simulink model "THERM_FMU"  (R2025b)
settings: Solver=FixedStepAuto  StartTime=0.0  StopTime=20  FixedStep=TsELEC  RelTol=1e-3  AbsTol=1e-6
values from neighbouring files (symbols this model uses):
  TsELEC = 5e-05    [initParams.mat]
  TsTHERMAL = 0.001    [initParams.mat]
undefined symbols (not defined in the file or in its folder): DiscIntNeverNeededParam
libraries: fl_lib x86, nesl_utility x29, SimscapeFluids_lib x4
(part 1 of 2)
Description:
  | Left Actuation System
settings Model: ExtModeAutoUpdateStatusClock=off  Creator=The MathWorks, Inc.  LastModifiedBy=gdudgeon
settings SolverCC: AutoScaleAbsTol=off  AlgebraicLoopSolver=TrustRegion
settings DataIOCC: ExternalInput=[]  InitialState=[]  SaveFormat=Array  SaveOutput=off  SaveTime=off
settings OptimizationCC: BlockReduction=off  BooleanDataType=off  InitFltsAndDblsToZero=on  BufferReusableBoundary=off
settings DebuggingCC: SaveWithParameterizedLinksMsg=none  SignalResolutionControl=TryResolveAllWithWarning  MultiTaskDSMMsg=warning  MultiTaskCondExecSysMsg=none  FcnCallInpInsideContextMsg=warning  UnconnectedInputMsg=warning  UnconnectedOutputMsg=warning  UnconnectedLineMsg=warning  BusObjectLabelMismatch=none  PregeneratedLibrarySubsystemCodeDiagnostic=none  SFUnexpectedBacktrackingDiag=warning  SFNoUnconditionalDefaultTransitionDiag=warning  SFExecutionAtInitializationDiag=none  ArithmeticOperatorsInVariantConditions=warning
settings HardwareCC: ProdBitPerPointer=32.0  ProdBitPerSizeT=32.0  ProdBitPerPtrDiffT=32.0  ProdLargestAtomicFloat=None  ProdIntDivRoundTo=Undefined  ProdEndianess=Unspecified  ProdWordSize=32.0  ProdHWDeviceType=32-bit Generic  TargetUnknown=on
settings ModelReferenceCC: EnableRefExpFcnMdlSchedulingChecks=on  PropagateSignalLabelsOutOfModel=off
settings SFSimCC: SimUseLocalCustomCode=off  CustomCodeUndefinedFunction=UseInterfaceOnly
settings RTWCC: RTWUseLocalCustomCode=off  GPUComputeCapability=3.5
settings CodeAppCC: StateflowObjectComments=on
settings GRTTargetCC: TargetLangStandard=C89/C90 (ANSI)
settings ConfigComp: CovMetricSettings=dw  CovSaveCumulativeToWorkspaceVar=on  CovSaveSingleToWorkspaceVar=on  CovExternalEMLEnable=off

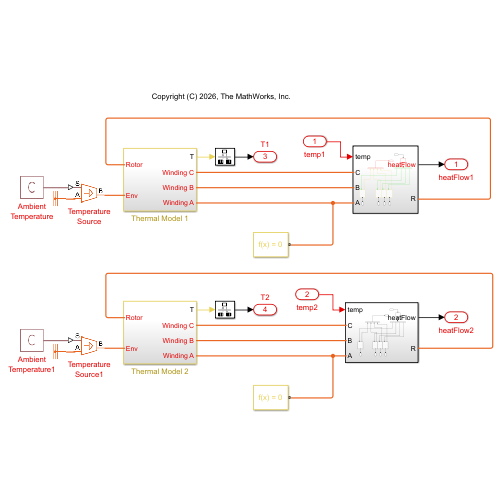
[thumbnail: Simulink's stored preview of the top-level diagram]
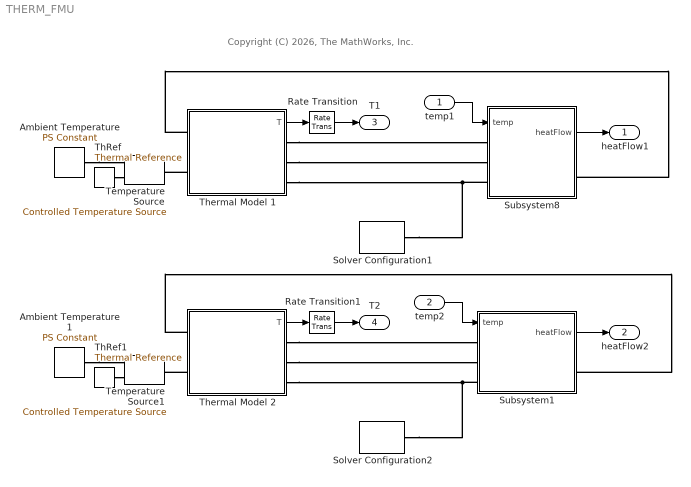
== system THERM_FMU ==
  note: Copyright (C) 2026, The MathWorks, Inc.
  temp1 : Inport  SampleTime=TsELEC
  temp2 : Inport  Port=2  SampleTime=TsELEC
  Ambient Temperature : fl_lib/Physical Signals/Sources/PS Constant  constant=300
  Ambient Temperature1 : fl_lib/Physical Signals/Sources/PS Constant  constant=300
  Rate Transition : RateTransition  OutPortSampleTime=TsELEC
  Rate Transition1 : RateTransition  OutPortSampleTime=TsELEC
  Solver Configuration1 : nesl_utility/Solver Configuration  PhysicalDomain=network_engine_domain  SubClassName=solver  LeftPortType=input  RightPortType=generic  Tones=[]  Harmonics=[]  SimulateNoise=off  Profile=off  UseLocalSampling=off  EnableSwitchedLinearOptims=on  FrequencyDomain=off  UseCCode=off  RelTol=0.001  AbsTol=1e-06  MinStep=1e-09  ToWorkspace=off  RevertToSquareIcSolve=off  NumHomotopyIterations=100  PhasorMode=off  PhasorModeNumHarmonics=1  ConsistencySolver=NEWTON_FTOL  IndexReductionMethod=DerivativeReplacement  DoDC=off  ResidualTolerance=1e-9  ConsistencyTolSource=GLOBAL  ConsistencyAbsTol=0.001  ConsistencyRelTol=0.001  ConsistencyTolFactor=0.001  UseLocalSolver=on  LocalSolverChoice=NE_BACKWARD_EULER_ADVANCER  ResolveIndetEquations=on  FunctionEvalNumThread=1  LocalSolverSampleTime=TsTHERMAL  DoFixedCost=on  MaxNonlinIter=1  MaxModeIter=2  ComputeImpulses=off  ImpulseIterations=2  LinearAlgebra=Full  LinearAlgebraNumThread=0  EquationFormulation=NE_TIME_EF  DelaysMemoryBudget=1024  AutomaticFiltering=on  FilteringTimeConstant=0.001  PartitionStorageMethod=AS_NEEDED  PartitionMemoryBudget=1024  PartitionMethod=FAST  MultibodyUseLocalSolver=off  MultibodyLocalSolverChoice=ODE1  MultibodyLocalSolverSampleTime=0.001
  Solver Configuration2 : nesl_utility/Solver Configuration  PhysicalDomain=network_engine_domain  SubClassName=solver  LeftPortType=input  RightPortType=generic  Tones=[]  Harmonics=[]  SimulateNoise=off  Profile=off  UseLocalSampling=off  EnableSwitchedLinearOptims=on  FrequencyDomain=off  UseCCode=off  RelTol=0.001  AbsTol=1e-06  MinStep=1e-09  ToWorkspace=off  RevertToSquareIcSolve=off  NumHomotopyIterations=100  PhasorMode=off  PhasorModeNumHarmonics=1  ConsistencySolver=NEWTON_FTOL  IndexReductionMethod=DerivativeReplacement  DoDC=off  ResidualTolerance=1e-9  ConsistencyTolSource=GLOBAL  ConsistencyAbsTol=0.001  ConsistencyRelTol=0.001  ConsistencyTolFactor=0.001  UseLocalSolver=on  LocalSolverChoice=NE_BACKWARD_EULER_ADVANCER  ResolveIndetEquations=on  FunctionEvalNumThread=1  LocalSolverSampleTime=TsTHERMAL  DoFixedCost=on  MaxNonlinIter=1  MaxModeIter=2  ComputeImpulses=off  ImpulseIterations=2  LinearAlgebra=Full  LinearAlgebraNumThread=0  EquationFormulation=NE_TIME_EF  DelaysMemoryBudget=1024  AutomaticFiltering=on  FilteringTimeConstant=0.001  PartitionStorageMethod=AS_NEEDED  PartitionMemoryBudget=1024  PartitionMethod=FAST  MultibodyUseLocalSolver=off  MultibodyLocalSolverChoice=ODE1  MultibodyLocalSolverSampleTime=0.001
  Subsystem1 : Subsystem
  Subsystem8 : Subsystem
  Temperature Source : fl_lib/Thermal/Thermal Sources/Controlled Temperature Source
  Temperature Source1 : fl_lib/Thermal/Thermal Sources/Controlled Temperature Source
  ThRef : fl_lib/Thermal/Thermal Elements/Thermal Reference
  ThRef1 : fl_lib/Thermal/Thermal Elements/Thermal Reference
  Thermal Model 1 : Subsystem  Tag=PublishSubsystem
  Thermal Model 2 : Subsystem  Tag=PublishSubsystem
  heatFlow1 : Outport  SampleTime=TsELEC
  heatFlow2 : Outport  Port=2  SampleTime=TsELEC
  T1 : Outport  Port=3  SampleTime=TsELEC
  T2 : Outport  Port=4  SampleTime=TsELEC
  wires:
  Subsystem8/1(heatFlow) -> heatFlow1/1
  temp2/1 -> Subsystem1/1(temp)
  Subsystem1/1(heatFlow) -> heatFlow2/1
  temp1/1 -> Subsystem8/1(temp)
  Thermal Model 1/1(T) -> Rate Transition/1
  Thermal Model 2/1(T) -> Rate Transition1/1
  Rate Transition/1 -> T1/1
  Rate Transition1/1 -> T2/1
  connections:
  Solver Configuration1/RConn1 -- Thermal Model 1/RConn3 -- Subsystem8/LConn3
  Subsystem1/LConn3 -- Thermal Model 2/RConn3 -- Solver Configuration2/RConn1
  ThRef1/LConn1 -- Temperature Source1/RConn2
  Thermal Model 2/RConn1 -- Subsystem1/LConn1
  ThRef/LConn1 -- Temperature Source/RConn2
  Thermal Model 2/LConn1 -- Subsystem1/RConn1
  Thermal Model 1/RConn2 -- Subsystem8/LConn2
  Ambient Temperature1/RConn1 -- Temperature Source1/RConn1
  Ambient Temperature/RConn1 -- Temperature Source/RConn1
  Thermal Model 1/RConn1 -- Subsystem8/LConn1
  Thermal Model 1/LConn1 -- Subsystem8/RConn1
  Thermal Model 2/RConn2 -- Subsystem1/LConn2
  Thermal Model 1/LConn2 -- Temperature Source/LConn1
  Thermal Model 2/LConn2 -- Temperature Source1/LConn1

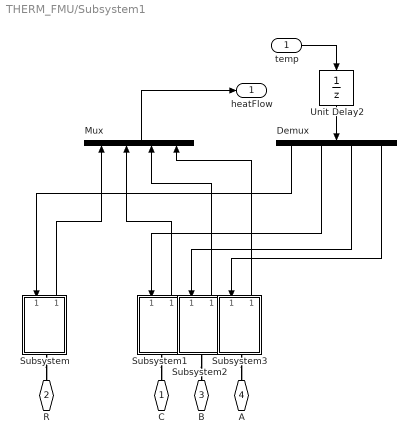
== system THERM_FMU/Subsystem1 ==
  temp : Inport
  Demux : Demux
  Mux : Mux
  Subsystem : Subsystem
      settings: PortSchema="{\"entries\":[{\"content\":{\"sides\":[{\"content\":{\"connectorIds\":[\"LConn1\"]},\"type\":\"ConnectorPlacement.EquallySpacedRectSide\",\"uuid\":\"9a881199-939f-4eef-aa67-0d9d87670dec\"},{\"content\":{\"connectorIds\":[\"In1\",\"Out1\"],\"side\":\"RIGHT\"},\"type\":\"ConnectorPlacement.EquallySpacedRectSide\",\"uuid\":\"59cd7e77-5157-4e0f-8bd7-0ab336b18f97\"},{\"content\":{\"connectorIds\":[],\"side\":\"TOP\"},\"type\":\"ConnectorPlacement.EquallySpacedRectSide\",\"uuid\":\"fe3b6155-18fe-4d88-946d-a6d9bcf9dc7a\"}]},\"type\":\"ConnectorPlacement.EquallySpacedConnector\",\"uuid\":\"f51b1317-3ac5-4211-9ee8-a1dae1b8baeb\"}],\"packageUris\":[\"http://schema.mathworks.com/mf0/Connector/19700101\"],\"version\":\"1.0\"}"
  Subsystem1 : Subsystem
      settings: PortSchema="{\"entries\":[{\"content\":{\"sides\":[{\"content\":{\"connectorIds\":[\"LConn1\"]},\"type\":\"ConnectorPlacement.EquallySpacedRectSide\",\"uuid\":\"9a881199-939f-4eef-aa67-0d9d87670dec\"},{\"content\":{\"connectorIds\":[\"In1\",\"Out1\"],\"side\":\"RIGHT\"},\"type\":\"ConnectorPlacement.EquallySpacedRectSide\",\"uuid\":\"59cd7e77-5157-4e0f-8bd7-0ab336b18f97\"},{\"content\":{\"connectorIds\":[],\"side\":\"TOP\"},\"type\":\"ConnectorPlacement.EquallySpacedRectSide\",\"uuid\":\"fe3b6155-18fe-4d88-946d-a6d9bcf9dc7a\"}]},\"type\":\"ConnectorPlacement.EquallySpacedConnector\",\"uuid\":\"f51b1317-3ac5-4211-9ee8-a1dae1b8baeb\"}],\"packageUris\":[\"http://schema.mathworks.com/mf0/Connector/19700101\"],\"version\":\"1.0\"}"
  Subsystem2 : Subsystem
      settings: PortSchema="{\"entries\":[{\"content\":{\"sides\":[{\"content\":{\"connectorIds\":[\"LConn1\"]},\"type\":\"ConnectorPlacement.EquallySpacedRectSide\",\"uuid\":\"9a881199-939f-4eef-aa67-0d9d87670dec\"},{\"content\":{\"connectorIds\":[\"In1\",\"Out1\"],\"side\":\"RIGHT\"},\"type\":\"ConnectorPlacement.EquallySpacedRectSide\",\"uuid\":\"59cd7e77-5157-4e0f-8bd7-0ab336b18f97\"},{\"content\":{\"connectorIds\":[],\"side\":\"TOP\"},\"type\":\"ConnectorPlacement.EquallySpacedRectSide\",\"uuid\":\"fe3b6155-18fe-4d88-946d-a6d9bcf9dc7a\"}]},\"type\":\"ConnectorPlacement.EquallySpacedConnector\",\"uuid\":\"f51b1317-3ac5-4211-9ee8-a1dae1b8baeb\"}],\"packageUris\":[\"http://schema.mathworks.com/mf0/Connector/19700101\"],\"version\":\"1.0\"}"
  Subsystem3 : Subsystem
      settings: PortSchema="{\"entries\":[{\"content\":{\"sides\":[{\"content\":{\"connectorIds\":[\"LConn1\"]},\"type\":\"ConnectorPlacement.EquallySpacedRectSide\",\"uuid\":\"9a881199-939f-4eef-aa67-0d9d87670dec\"},{\"content\":{\"connectorIds\":[\"In1\",\"Out1\"],\"side\":\"RIGHT\"},\"type\":\"ConnectorPlacement.EquallySpacedRectSide\",\"uuid\":\"59cd7e77-5157-4e0f-8bd7-0ab336b18f97\"},{\"content\":{\"connectorIds\":[],\"side\":\"TOP\"},\"type\":\"ConnectorPlacement.EquallySpacedRectSide\",\"uuid\":\"fe3b6155-18fe-4d88-946d-a6d9bcf9dc7a\"}]},\"type\":\"ConnectorPlacement.EquallySpacedConnector\",\"uuid\":\"f51b1317-3ac5-4211-9ee8-a1dae1b8baeb\"}],\"packageUris\":[\"http://schema.mathworks.com/mf0/Connector/19700101\"],\"version\":\"1.0\"}"
  Unit Delay2 : UnitDelay  InitialCondition=323.15  SampleTime=TsELEC  HasFrameUpgradeWarning=on
  C : PMIOPort  Side=Left
  R : PMIOPort  Port=2  Side=Right
  B : PMIOPort  Port=3  Side=Left
  A : PMIOPort  Port=4  Side=Left
  heatFlow : Outport  SampleTime=TsELEC
  wires:
  temp/1 -> Unit Delay2/1
  Mux/1 -> heatFlow/1
  Subsystem3/1(heatFlow) -> Mux/4
  Demux/4 -> Subsystem3/1(temp)
  Subsystem/1(heatFlow) -> Mux/1
  Demux/1 -> Subsystem/1(temp)
  Unit Delay2/1 -> Demux/1
  Subsystem2/1(heatFlow) -> Mux/3
  Subsystem1/1(heatFlow) -> Mux/2
  Demux/3 -> Subsystem2/1(temp)
  Demux/2 -> Subsystem1/1(temp)
  connections:
  Subsystem1/LConn1 -- C/RConn1
  Subsystem/LConn1 -- R/RConn1
  Subsystem3/LConn1 -- A/RConn1
  Subsystem2/LConn1 -- B/RConn1

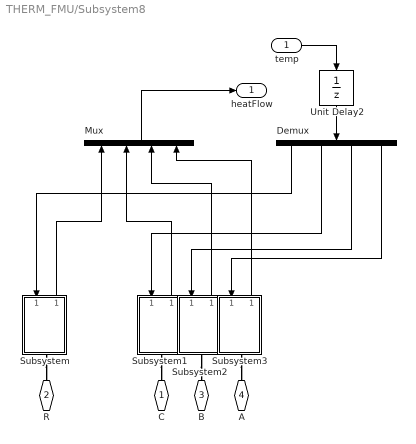
== system THERM_FMU/Subsystem8 ==
  temp : Inport
  Demux : Demux
  Mux : Mux
  Subsystem : Subsystem
      settings: PortSchema="{\"entries\":[{\"content\":{\"sides\":[{\"content\":{\"connectorIds\":[\"LConn1\"]},\"type\":\"ConnectorPlacement.EquallySpacedRectSide\",\"uuid\":\"9a881199-939f-4eef-aa67-0d9d87670dec\"},{\"content\":{\"connectorIds\":[\"In1\",\"Out1\"],\"side\":\"RIGHT\"},\"type\":\"ConnectorPlacement.EquallySpacedRectSide\",\"uuid\":\"59cd7e77-5157-4e0f-8bd7-0ab336b18f97\"},{\"content\":{\"connectorIds\":[],\"side\":\"TOP\"},\"type\":\"ConnectorPlacement.EquallySpacedRectSide\",\"uuid\":\"fe3b6155-18fe-4d88-946d-a6d9bcf9dc7a\"}]},\"type\":\"ConnectorPlacement.EquallySpacedConnector\",\"uuid\":\"f51b1317-3ac5-4211-9ee8-a1dae1b8baeb\"}],\"packageUris\":[\"http://schema.mathworks.com/mf0/Connector/19700101\"],\"version\":\"1.0\"}"
  Subsystem1 : Subsystem
      settings: PortSchema="{\"entries\":[{\"content\":{\"sides\":[{\"content\":{\"connectorIds\":[\"LConn1\"]},\"type\":\"ConnectorPlacement.EquallySpacedRectSide\",\"uuid\":\"9a881199-939f-4eef-aa67-0d9d87670dec\"},{\"content\":{\"connectorIds\":[\"In1\",\"Out1\"],\"side\":\"RIGHT\"},\"type\":\"ConnectorPlacement.EquallySpacedRectSide\",\"uuid\":\"59cd7e77-5157-4e0f-8bd7-0ab336b18f97\"},{\"content\":{\"connectorIds\":[],\"side\":\"TOP\"},\"type\":\"ConnectorPlacement.EquallySpacedRectSide\",\"uuid\":\"fe3b6155-18fe-4d88-946d-a6d9bcf9dc7a\"}]},\"type\":\"ConnectorPlacement.EquallySpacedConnector\",\"uuid\":\"f51b1317-3ac5-4211-9ee8-a1dae1b8baeb\"}],\"packageUris\":[\"http://schema.mathworks.com/mf0/Connector/19700101\"],\"version\":\"1.0\"}"
  Subsystem2 : Subsystem
      settings: PortSchema="{\"entries\":[{\"content\":{\"sides\":[{\"content\":{\"connectorIds\":[\"LConn1\"]},\"type\":\"ConnectorPlacement.EquallySpacedRectSide\",\"uuid\":\"9a881199-939f-4eef-aa67-0d9d87670dec\"},{\"content\":{\"connectorIds\":[\"In1\",\"Out1\"],\"side\":\"RIGHT\"},\"type\":\"ConnectorPlacement.EquallySpacedRectSide\",\"uuid\":\"59cd7e77-5157-4e0f-8bd7-0ab336b18f97\"},{\"content\":{\"connectorIds\":[],\"side\":\"TOP\"},\"type\":\"ConnectorPlacement.EquallySpacedRectSide\",\"uuid\":\"fe3b6155-18fe-4d88-946d-a6d9bcf9dc7a\"}]},\"type\":\"ConnectorPlacement.EquallySpacedConnector\",\"uuid\":\"f51b1317-3ac5-4211-9ee8-a1dae1b8baeb\"}],\"packageUris\":[\"http://schema.mathworks.com/mf0/Connector/19700101\"],\"version\":\"1.0\"}"
  Subsystem3 : Subsystem
      settings: PortSchema="{\"entries\":[{\"content\":{\"sides\":[{\"content\":{\"connectorIds\":[\"LConn1\"]},\"type\":\"ConnectorPlacement.EquallySpacedRectSide\",\"uuid\":\"9a881199-939f-4eef-aa67-0d9d87670dec\"},{\"content\":{\"connectorIds\":[\"In1\",\"Out1\"],\"side\":\"RIGHT\"},\"type\":\"ConnectorPlacement.EquallySpacedRectSide\",\"uuid\":\"59cd7e77-5157-4e0f-8bd7-0ab336b18f97\"},{\"content\":{\"connectorIds\":[],\"side\":\"TOP\"},\"type\":\"ConnectorPlacement.EquallySpacedRectSide\",\"uuid\":\"fe3b6155-18fe-4d88-946d-a6d9bcf9dc7a\"}]},\"type\":\"ConnectorPlacement.EquallySpacedConnector\",\"uuid\":\"f51b1317-3ac5-4211-9ee8-a1dae1b8baeb\"}],\"packageUris\":[\"http://schema.mathworks.com/mf0/Connector/19700101\"],\"version\":\"1.0\"}"
  Unit Delay2 : UnitDelay  InitialCondition=323.15  SampleTime=TsELEC  HasFrameUpgradeWarning=on
  C : PMIOPort  Side=Left
  R : PMIOPort  Port=2  Side=Right
  B : PMIOPort  Port=3  Side=Left
  A : PMIOPort  Port=4  Side=Left
  heatFlow : Outport  SampleTime=TsELEC
  wires:
  Demux/2 -> Subsystem1/1(temp)
  Demux/3 -> Subsystem2/1(temp)
  Subsystem1/1(heatFlow) -> Mux/2
  Subsystem2/1(heatFlow) -> Mux/3
  Unit Delay2/1 -> Demux/1
  Demux/1 -> Subsystem/1(temp)
  Subsystem/1(heatFlow) -> Mux/1
  Demux/4 -> Subsystem3/1(temp)
  Subsystem3/1(heatFlow) -> Mux/4
  Mux/1 -> heatFlow/1
  temp/1 -> Unit Delay2/1
  connections:
  Subsystem2/LConn1 -- B/RConn1
  Subsystem3/LConn1 -- A/RConn1
  Subsystem/LConn1 -- R/RConn1
  Subsystem1/LConn1 -- C/RConn1

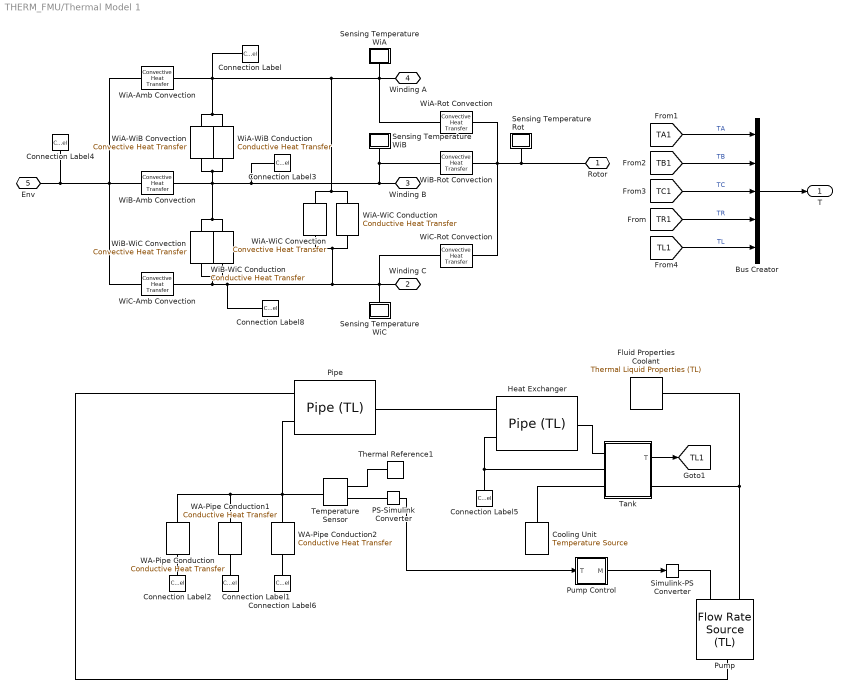
== system THERM_FMU/Thermal Model 1 ==
  Bus Creator : BusCreator  Inputs=5
  Connection Label : ConnectionLabel  Label=WindingA
  Connection Label1 : ConnectionLabel  Label=WindingB
  Connection Label2 : ConnectionLabel  Label=WindingA
  Connection Label3 : ConnectionLabel  Label=WindingB
  Connection Label4 : ConnectionLabel  Label=Env
  Connection Label5 : ConnectionLabel  Label=Env
  Connection Label6 : ConnectionLabel  Label=WindingC
  Connection Label8 : ConnectionLabel  Label=WindingC
  Cooling Unit : fl_lib/Thermal/Thermal Sources/Temperature Source  temperature=278 K
  "Fluid Properties Coolant " : SimscapeFluids_lib/Thermal Liquid/Utilities/Thermal Liquid Properties (TL)  fluid_list=fluids.thermal_liquid.utilities.enum.thermal_liquid_fluid_list.ethylene_glycol  concentration_param_EG=fluids.thermal_liquid.utilities.enum.thermal_liquid_concentration.volume_fraction  concentration_param_PG=fluids.thermal_liquid.utilities.enum.thermal_liquid_concentration.volume_fraction  c_mass_SW=3.5e-3  c_mass_EG=0.1  c_mass_PG=0.1  c_mass_GL=0.1  c_vol_EG=0.1  c_vol_PG=0.1  beta_const_EG=2.1791 GPa  beta_const_PG=2.1791 GPa  beta_const_GL=2.1791 GPa  p_min_EG=0.01 MPa  p_min_PG=0.01 MPa  p_min_GL=0.01 MPa  p_max_EG=50 MPa  p_max_PG=50 MPa  p_max_GL=50 MPa  p_atm=0.101325 MPa  properties_range_check=simscape.enum.assert.action.error
  Heat Exchanger : SimscapeFluids_lib/Thermal Liquid/Pipes & Fittings/Pipe (TL)  dynamic_compressibility=0  inertia=0  num_segments=1  pipe_length=10 m  cross_section_geometry=fluids.thermal_liquid.pipes_fittings.enum.CrossSectionGeometry.Custom  pipe_diameter=0.1 m  pipe_inner_diameter=0.05 m  pipe_outer_diameter=0.1 m  pipe_width=0.1 m  pipe_height=0.1 m  pipe_major_axis=0.1 m  pipe_minor_axis=0.05 m  pipe_side=0.1 m  pipe_angle=30 deg  area=0.01^2/4*pi m^2  Dh=0.1128 m  elevation_spec=foundation.enum.constant_variable.constant  elevation_gain=0 m  gravity_spec=foundation.enum.constant_variable.constant  g=9.81 m/s^2  pressure_loss_spec=1  local_pressure_loss_spec=fluids.thermal_liquid.pipes_fittings.enum.LocalLossSpec.AggregateLength  length_add=0.1 m  loss_coefficient=0.1  roughness_spec=fluids.thermal_liquid.pipes_fittings.enum.RoughnessSpec.Custom  roughness=1.5e-5 m  Re_friction_TLU=[ 400 1000 1.5e+3 3e+3 4e+3 6e+3 1e+4 2e+4 4e+4 6e+4 1e+5 1e+8 ]  friction_factor_TLU=[ 0.264 0.112 0.07099999999999999 0.0417 0.0387 0.0268 0.025 0.0232 0.0226 0.022 0.0214 0.0214 ]  Re_lam=2e+3  Re_tur=4e+3  shape_factor=64  mdot_nominal=[ 0.1 1 ] kg/s  p_diff_nominal=[ 0.001 0.01 ] MPa  mdot_threshold=1e-6 kg/s  wall_spec=1  vol_expansion_spec=fluids.thermal_liquid.pipes_fittings.enum.VolumeExpansionSpec.Diameter  area_pressure_gain=1e-6 m^2/MPa  static_pressure_TLU=[.1, 1] MPa  area_pressure_gain_TLU=[1e-05, 1.1e-05] m^2  material_behavior_spec=fluids.thermal_liquid.pipes_fittings.enum.PipeMaterialBehavior.Linear  diameter_pressure_gain=1.2e-6 m/MPa  wall_thickness=0.05 m  elastic_modulus=69 GPa  stress_TLU=[276, 310] MPa  strain_TLU=[.004, .02]  stress_assert_action=simscape.enum.assert.action.none  stress_max=400 MPa  poisson_ratio=0.33  wall_time_constant=0.01 s  thermal_expansion=false  alpha_L_wall=24 um/(deltaK*m)  thermal_expansion_Tref=293.15 K  heat_transfer_spec=1  mdot_nominal_heat=[ 0.1 1 ] kg/s  T_in_nominal=[ 293.15 293.15 ] K  T_out_nominal=[ 300 300 ] K  p_in_nominal_heat=[ 0.101325 0.101325 ] MPa  T_wall_nominal=[ 303.15 303.15 ] K  a_coeff=0.023  b_Re_power=0.8  c_Pr_power=0.4  Nu_lam=3.66  Re_Colburn_TLU=[ 100 150 1000 ]  Colburn_factor_TLU=[ 0.019 0.013 0.002 ]  Re_Nu_TLU=[ 100 150 1000 ]  Pr_Nu_TLU=[ 1 10 ]  Nu_TLU=[ 3.72 4.21; 3.75 4.44; 4.21 7.15 ]  p0_vec=0.101325 MPa  T0_vec=300 K  mdot0=0.1 kg/s  p_nominal=0.101325 MPa  T_nominal=293.15 K
  PS-Simulink Converter : nesl_utility/PS-Simulink Converter  PhysicalDomain=network_engine_domain  SubClassName=ps_output  LeftPortType=input  RightPortType=output  PseudoPeriodic=off  Frequencies=[]  VectorFormat=1-D array  Unit=inherit  AffineConversion=off
  Pipe : SimscapeFluids_lib/Thermal Liquid/Pipes & Fittings/Pipe (TL)  dynamic_compressibility=0  inertia=0  num_segments=1  pipe_length=1 m  cross_section_geometry=fluids.thermal_liquid.pipes_fittings.enum.CrossSectionGeometry.Custom  pipe_diameter=0.1 m  pipe_inner_diameter=0.05 m  pipe_outer_diameter=0.1 m  pipe_width=0.1 m  pipe_height=0.1 m  pipe_major_axis=0.1 m  pipe_minor_axis=0.05 m  pipe_side=0.1 m  pipe_angle=30 deg  area=0.01^2/4*pi m^2  Dh=0.1128 m  elevation_spec=foundation.enum.constant_variable.constant  elevation_gain=0 m  gravity_spec=foundation.enum.constant_variable.constant  g=9.81 m/s^2  pressure_loss_spec=1  local_pressure_loss_spec=fluids.thermal_liquid.pipes_fittings.enum.LocalLossSpec.AggregateLength  length_add=0.1 m  loss_coefficient=0.1  roughness_spec=fluids.thermal_liquid.pipes_fittings.enum.RoughnessSpec.Custom  roughness=1.5e-5 m  Re_friction_TLU=[ 400 1000 1.5e+3 3e+3 4e+3 6e+3 1e+4 2e+4 4e+4 6e+4 1e+5 1e+8 ]  friction_factor_TLU=[ 0.264 0.112 0.07099999999999999 0.0417 0.0387 0.0268 0.025 0.0232 0.0226 0.022 0.0214 0.0214 ]  Re_lam=2e+3  Re_tur=4e+3  shape_factor=64  mdot_nominal=[ 0.1 1 ] kg/s  p_diff_nominal=[ 0.001 0.01 ] MPa  mdot_threshold=1e-6 kg/s  wall_spec=1  vol_expansion_spec=fluids.thermal_liquid.pipes_fittings.enum.VolumeExpansionSpec.Diameter  area_pressure_gain=1e-6 m^2/MPa  static_pressure_TLU=[.1, 1] MPa  area_pressure_gain_TLU=[1e-05, 1.1e-05] m^2  material_behavior_spec=fluids.thermal_liquid.pipes_fittings.enum.PipeMaterialBehavior.Linear  diameter_pressure_gain=1.2e-6 m/MPa  wall_thickness=0.05 m  elastic_modulus=69 GPa  stress_TLU=[276, 310] MPa  strain_TLU=[.004, .02]  stress_assert_action=simscape.enum.assert.action.none  stress_max=400 MPa  poisson_ratio=0.33  wall_time_constant=0.01 s  thermal_expansion=false  alpha_L_wall=24 um/(deltaK*m)  thermal_expansion_Tref=293.15 K  heat_transfer_spec=1  mdot_nominal_heat=[ 0.1 1 ] kg/s  T_in_nominal=[ 293.15 293.15 ] K  T_out_nominal=[ 300 300 ] K  p_in_nominal_heat=[ 0.101325 0.101325 ] MPa  T_wall_nominal=[ 303.15 303.15 ] K  a_coeff=0.023  b_Re_power=0.8  c_Pr_power=0.4  Nu_lam=3.66  Re_Colburn_TLU=[ 100 150 1000 ]  Colburn_factor_TLU=[ 0.019 0.013 0.002 ]  Re_Nu_TLU=[ 100 150 1000 ]  Pr_Nu_TLU=[ 1 10 ]  Nu_TLU=[ 3.72 4.21; 3.75 4.44; 4.21 7.15 ]  p0_vec=0.101325 MPa  T0_vec=300 K  mdot0=0.1 kg/s  p_nominal=0.101325 MPa  T_nominal=293.15 K
  Pump : fl_lib/Thermal Liquid/Sources/Flow Rate Source (TL)  source_type=foundation.enum.constant_controlled.controlled  flow_type=foundation.enum.mass_volumetric_flow.mass  mass_flow=0 kg/s  volumetric_flow=0 m^3/s  power_spec=foundation.enum.power_spec.isentropic  area=0.01^2/4*pi m^2
  Pump Control : Subsystem
  Sensing Temperature Rot : Subsystem
      mask Display: disp('TR')
  Sensing Temperature WiA : Subsystem
      mask Display: disp('TA')
  Sensing Temperature WiB : Subsystem
      mask Display: disp('TB')
  Sensing Temperature WiC : Subsystem
      mask Display: disp('TC')
  Simulink-PS Converter : nesl_utility/Simulink-PS Converter  PhysicalDomain=network_engine_domain  SubClassName=ps_input  LeftPortType=input  RightPortType=output  PseudoPeriodic=off  Frequencies=[]  NoiseDistribution=none  NoiseParameters=[]  Unit=1  AffineConversion=off  FilteringAndDerivatives=provide  SimscapeFilterOrder=1  InputFilterTimeConstant=0.001  UdotUserProvided=0
  Tank : Subsystem
  Temperature Sensor : fl_lib/Thermal/Thermal Sensors/Temperature Sensor  temperature_measure=foundation.enum.MeasurementReference.difference
  Thermal Reference1 : fl_lib/Thermal/Thermal Elements/Thermal Reference
  WA-Pipe Conduction : fl_lib/Thermal/Thermal Elements/Conductive Heat Transfer  thermal_type=foundation.enum.ConstantVariableTabulated.Constant  wall_geometry=foundation.enum.ConductionWallGeometry.Planar  area=0.1 m^2  thickness=0.1 m  d_in=0.05 m  d_out=0.1 m  L=1 m  th_cond_min=10 W/(K*m)  th_cond=80 W/(m*K)  th_cond_TLU=[413, 401, 392, 383, 371, 357, 342] W/(K*m)  temp_TLU=[200, 273, 400, 600, 800, 1000, 1200] K  T_specify=off  T_priority=None  T=0 K  T_nominal_specify=off  T_nominal_value=1  T_nominal_unit=K  Q_specify=off  Q_priority=None  Q=0 J/s  Q_nominal_specify=off  Q_nominal_value=1  Q_nominal_unit=J/s
  WA-Pipe Conduction1 : fl_lib/Thermal/Thermal Elements/Conductive Heat Transfer  thermal_type=foundation.enum.ConstantVariableTabulated.Constant  wall_geometry=foundation.enum.ConductionWallGeometry.Planar  area=0.1 m^2  thickness=0.1 m  d_in=0.05 m  d_out=0.1 m  L=1 m  th_cond_min=10 W/(K*m)  th_cond=80 W/(m*K)  th_cond_TLU=[413, 401, 392, 383, 371, 357, 342] W/(K*m)  temp_TLU=[200, 273, 400, 600, 800, 1000, 1200] K  T_specify=off  T_priority=None  T=0 K  T_nominal_specify=off  T_nominal_value=1  T_nominal_unit=K  Q_specify=off  Q_priority=None  Q=0 J/s  Q_nominal_specify=off  Q_nominal_value=1  Q_nominal_unit=J/s
  WA-Pipe Conduction2 : fl_lib/Thermal/Thermal Elements/Conductive Heat Transfer  thermal_type=foundation.enum.ConstantVariableTabulated.Constant  wall_geometry=foundation.enum.ConductionWallGeometry.Planar  area=0.1 m^2  thickness=0.1 m  d_in=0.05 m  d_out=0.1 m  L=1 m  th_cond_min=10 W/(K*m)  th_cond=80 W/(m*K)  th_cond_TLU=[413, 401, 392, 383, 371, 357, 342] W/(K*m)  temp_TLU=[200, 273, 400, 600, 800, 1000, 1200] K  T_specify=off  T_priority=None  T=0 K  T_nominal_specify=off  T_nominal_value=1  T_nominal_unit=K  Q_specify=off  Q_priority=None  Q=0 J/s  Q_nominal_specify=off  Q_nominal_value=1  Q_nominal_unit=J/s
  WiA-Amb Convection : fl_lib/Thermal/Thermal Elements/Convective Heat Transfer  thermal_type=foundation.enum.constant_variable.constant  area=1 m^2  heat_tr_coeff=0.1 W/(m^2 * K)  min_heat_tr_coeff=1e-3 W/(K*m^2)  T_specify=off  T_priority=None  T=0 K  T_nominal_specify=off  T_nominal_value=1  T_nominal_unit=K  Q_specify=off  Q_priority=None  Q=0 J/s  Q_nominal_specify=off  Q_nominal_value=1  Q_nominal_unit=J/s
  WiA-Rot Convection : fl_lib/Thermal/Thermal Elements/Convective Heat Transfer  thermal_type=foundation.enum.constant_variable.constant  area=1 m^2  heat_tr_coeff=0.1 W/(m^2 * K)  min_heat_tr_coeff=1e-3 W/(K*m^2)  T_specify=off  T_priority=None  T=0 K  T_nominal_specify=off  T_nominal_value=1  T_nominal_unit=K  Q_specify=off  Q_priority=None  Q=0 J/s  Q_nominal_specify=off  Q_nominal_value=1  Q_nominal_unit=J/s
  WiA-WiB Conduction : fl_lib/Thermal/Thermal Elements/Conductive Heat Transfer  thermal_type=foundation.enum.ConstantVariableTabulated.Constant  wall_geometry=foundation.enum.ConductionWallGeometry.Planar  area=1 m^2  thickness=1 m  d_in=0.05 m  d_out=0.1 m  L=1 m  th_cond_min=10 W/(K*m)  th_cond=0.1 W/(m*K)  th_cond_TLU=[413, 401, 392, 383, 371, 357, 342] W/(K*m)  temp_TLU=[200, 273, 400, 600, 800, 1000, 1200] K  T_specify=off  T_priority=None  T=0 K  T_nominal_specify=off  T_nominal_value=1  T_nominal_unit=K  Q_specify=off  Q_priority=None  Q=0 J/s  Q_nominal_specify=off  Q_nominal_value=1  Q_nominal_unit=J/s
  WiA-WiB Convection : fl_lib/Thermal/Thermal Elements/Convective Heat Transfer  thermal_type=foundation.enum.constant_variable.constant  area=1 m^2  heat_tr_coeff=0.1 W/(m^2 * K)  min_heat_tr_coeff=1e-3 W/(K*m^2)  T_specify=off  T_priority=None  T=0 K  T_nominal_specify=off  T_nominal_value=1  T_nominal_unit=K  Q_specify=off  Q_priority=None  Q=0 J/s  Q_nominal_specify=off  Q_nominal_value=1  Q_nominal_unit=J/s
  WiA-WiC Conduction : fl_lib/Thermal/Thermal Elements/Conductive Heat Transfer  thermal_type=foundation.enum.ConstantVariableTabulated.Constant  wall_geometry=foundation.enum.ConductionWallGeometry.Planar  area=1 m^2  thickness=1 m  d_in=0.05 m  d_out=0.1 m  L=1 m  th_cond_min=10 W/(K*m)  th_cond=0.1 W/(m*K)  th_cond_TLU=[413, 401, 392, 383, 371, 357, 342] W/(K*m)  temp_TLU=[200, 273, 400, 600, 800, 1000, 1200] K  T_specify=off  T_priority=None  T=0 K  T_nominal_specify=off  T_nominal_value=1  T_nominal_unit=K  Q_specify=off  Q_priority=None  Q=0 J/s  Q_nominal_specify=off  Q_nominal_value=1  Q_nominal_unit=J/s
  WiA-WiC Convection : fl_lib/Thermal/Thermal Elements/Convective Heat Transfer  thermal_type=foundation.enum.constant_variable.constant  area=1 m^2  heat_tr_coeff=0.1 W/(m^2 * K)  min_heat_tr_coeff=1e-3 W/(K*m^2)  T_specify=off  T_priority=None  T=0 K  T_nominal_specify=off  T_nominal_value=1  T_nominal_unit=K  Q_specify=off  Q_priority=None  Q=0 J/s  Q_nominal_specify=off  Q_nominal_value=1  Q_nominal_unit=J/s
  WiB-Amb Convection : fl_lib/Thermal/Thermal Elements/Convective Heat Transfer  thermal_type=foundation.enum.constant_variable.constant  area=1 m^2  heat_tr_coeff=0.1 W/(m^2 * K)  min_heat_tr_coeff=1e-3 W/(K*m^2)  T_specify=off  T_priority=None  T=0 K  T_nominal_specify=off  T_nominal_value=1  T_nominal_unit=K  Q_specify=off  Q_priority=None  Q=0 J/s  Q_nominal_specify=off  Q_nominal_value=1  Q_nominal_unit=J/s
  WiB-Rot Convection : fl_lib/Thermal/Thermal Elements/Convective Heat Transfer  thermal_type=foundation.enum.constant_variable.constant  area=1 m^2  heat_tr_coeff=0.1 W/(m^2 * K)  min_heat_tr_coeff=1e-3 W/(K*m^2)  T_specify=off  T_priority=None  T=0 K  T_nominal_specify=off  T_nominal_value=1  T_nominal_unit=K  Q_specify=off  Q_priority=None  Q=0 J/s  Q_nominal_specify=off  Q_nominal_value=1  Q_nominal_unit=J/s
  WiB-WiC Conduction : fl_lib/Thermal/Thermal Elements/Conductive Heat Transfer  thermal_type=foundation.enum.ConstantVariableTabulated.Constant  wall_geometry=foundation.enum.ConductionWallGeometry.Planar  area=1 m^2  thickness=1 m  d_in=0.05 m  d_out=0.1 m  L=1 m  th_cond_min=10 W/(K*m)  th_cond=0.1 W/(m*K)  th_cond_TLU=[413, 401, 392, 383, 371, 357, 342] W/(K*m)  temp_TLU=[200, 273, 400, 600, 800, 1000, 1200] K  T_specify=off  T_priority=None  T=0 K  T_nominal_specify=off  T_nominal_value=1  T_nominal_unit=K  Q_specify=off  Q_priority=None  Q=0 J/s  Q_nominal_specify=off  Q_nominal_value=1  Q_nominal_unit=J/s
  WiB-WiC Convection : fl_lib/Thermal/Thermal Elements/Convective Heat Transfer  thermal_type=foundation.enum.constant_variable.constant  area=1 m^2  heat_tr_coeff=0.1 W/(m^2 * K)  min_heat_tr_coeff=1e-3 W/(K*m^2)  T_specify=off  T_priority=None  T=0 K  T_nominal_specify=off  T_nominal_value=1  T_nominal_unit=K  Q_specify=off  Q_priority=None  Q=0 J/s  Q_nominal_specify=off  Q_nominal_value=1  Q_nominal_unit=J/s
  WiC-Amb Convection : fl_lib/Thermal/Thermal Elements/Convective Heat Transfer  thermal_type=foundation.enum.constant_variable.constant  area=1 m^2  heat_tr_coeff=0.1 W/(m^2 * K)  min_heat_tr_coeff=1e-3 W/(K*m^2)  T_specify=off  T_priority=None  T=0 K  T_nominal_specify=off  T_nominal_value=1  T_nominal_unit=K  Q_specify=off  Q_priority=None  Q=0 J/s  Q_nominal_specify=off  Q_nominal_value=1  Q_nominal_unit=J/s
  WiC-Rot Convection : fl_lib/Thermal/Thermal Elements/Convective Heat Transfer  thermal_type=foundation.enum.constant_variable.constant  area=1 m^2  heat_tr_coeff=0.1 W/(m^2 * K)  min_heat_tr_coeff=1e-3 W/(K*m^2)  T_specify=off  T_priority=None  T=0 K  T_nominal_specify=off  T_nominal_value=1  T_nominal_unit=K  Q_specify=off  Q_priority=None  Q=0 J/s  Q_nominal_specify=off  Q_nominal_value=1  Q_nominal_unit=J/s
  Rotor : PMIOPort  Side=Left
  Winding C : PMIOPort  Port=2  Side=Right
  Winding B : PMIOPort  Port=3  Side=Right
  Winding A : PMIOPort  Port=4  Side=Right
  Env : PMIOPort  Port=5  Side=Left
  T : Outport
  tag scope: TL1=global
  wires:
  Pump Control/1(M) -> Simulink-PS Converter/1
  PS-Simulink Converter/1 -> Pump Control/1(T)
  Tank/1(T) -> [TL1]
  [TL1] -> Bus Creator/5  "TL"
  [TR1] -> Bus Creator/4  "TR"
  [TC1] -> Bus Creator/3  "TC"
  [TB1] -> Bus Creator/2  "TB"
  [TA1] -> Bus Creator/1  "TA"
  Bus Creator/1 -> T/1
  connections:
  Pipe/LConn1 -- Pump/RConn1
  WA-Pipe Conduction/LConn1 -- Connection Label2/LConn1
  Simulink-PS Converter/RConn1 -- Pump/LConn2
  Heat Exchanger/LConn1 -- Pipe/RConn1
  Tank/LConn1 -- Heat Exchanger/RConn1
  WA-Pipe Conduction1/LConn1 -- Connection Label1/LConn1
  WA-Pipe Conduction2/LConn1 -- Connection Label6/LConn1
  Thermal Reference1/LConn1 -- Temperature Sensor/RConn1
  Tank/LConn3 -- Cooling Unit/LConn1
  PS-Simulink Converter/LConn1 -- Temperature Sensor/RConn2
  Tank/LConn2 -- Connection Label5/LConn1 -- Heat Exchanger/LConn2
  Tank/RConn1 -- Pump/LConn1 -- "Fluid Properties Coolant "/RConn1
  WA-Pipe Conduction1/RConn1 -- Pipe/LConn2 -- WA-Pipe Conduction2/RConn1 -- Temperature Sensor/LConn1 -- WA-Pipe Conduction/RConn1
  Sensing Temperature Rot/LConn1 -- Rotor/RConn1 -- WiC-Rot Convection/LConn1 -- WiB-Rot Convection/LConn1 -- WiA-Rot Convection/LConn1
  WiA-Rot Convection/RConn1 -- WiA-WiC Conduction/RConn1 -- WiA-WiC Convection/RConn1 -- WiA-WiB Convection/LConn1 -- WiA-WiB Conduction/LConn1 -- WiA-Amb Convection/LConn1 -- Connection Label/LConn1 -- Sensing Temperature WiA/LConn1 -- Winding A/RConn1
  WiA-WiB Convection/RConn1 -- WiA-WiB Conduction/RConn1 -- WiB-Amb Convection/LConn1 -- Sensing Temperature WiB/LConn1 -- WiB-Rot Convection/RConn1 -- Winding B/RConn1 -- Connection Label3/LConn1 -- WiB-WiC Conduction/LConn1 -- WiB-WiC Convection/LConn1
  WiC-Rot Convection/RConn1 -- Winding C/RConn1 -- WiB-WiC Conduction/RConn1 -- WiB-WiC Convection/RConn1 -- WiC-Amb Convection/LConn1 -- Connection Label8/LConn1 -- WiA-WiC Convection/LConn1 -- WiA-WiC Conduction/LConn1 -- Sensing Temperature WiC/LConn1
  WiA-Amb Convection/RConn1 -- WiC-Amb Convection/RConn1 -- Env/RConn1 -- Connection Label4/LConn1 -- WiB-Amb Convection/RConn1

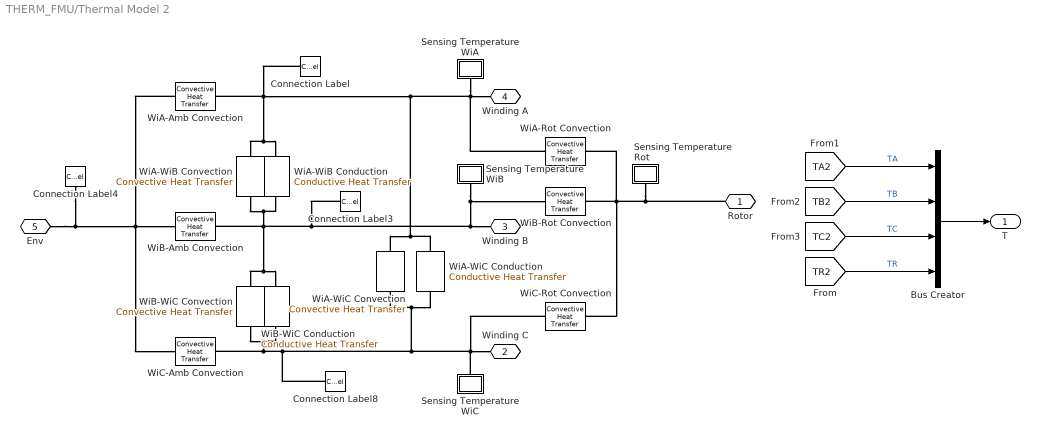
== system THERM_FMU/Thermal Model 2 ==
  Bus Creator : BusCreator  Inputs=4
  Connection Label : ConnectionLabel  Label=WindingA
  Connection Label3 : ConnectionLabel  Label=WindingB
  Connection Label4 : ConnectionLabel  Label=Env
  Connection Label8 : ConnectionLabel  Label=WindingC
  Sensing Temperature Rot : Subsystem
      mask Display: disp('TR')
  Sensing Temperature WiA : Subsystem
      mask Display: disp('TA')
  Sensing Temperature WiB : Subsystem
      mask Display: disp('TB')
  Sensing Temperature WiC : Subsystem
      mask Display: disp('TC')
  WiA-Amb Convection : fl_lib/Thermal/Thermal Elements/Convective Heat Transfer  thermal_type=foundation.enum.constant_variable.constant  area=1 m^2  heat_tr_coeff=0.1 W/(m^2 * K)  min_heat_tr_coeff=1e-3 W/(K*m^2)  T_specify=off  T_priority=None  T=0 K  T_nominal_specify=off  T_nominal_value=1  T_nominal_unit=K  Q_specify=off  Q_priority=None  Q=0 J/s  Q_nominal_specify=off  Q_nominal_value=1  Q_nominal_unit=J/s
  WiA-Rot Convection : fl_lib/Thermal/Thermal Elements/Convective Heat Transfer  thermal_type=foundation.enum.constant_variable.constant  area=1 m^2  heat_tr_coeff=0.1 W/(m^2 * K)  min_heat_tr_coeff=1e-3 W/(K*m^2)  T_specify=off  T_priority=None  T=0 K  T_nominal_specify=off  T_nominal_value=1  T_nominal_unit=K  Q_specify=off  Q_priority=None  Q=0 J/s  Q_nominal_specify=off  Q_nominal_value=1  Q_nominal_unit=J/s
  WiA-WiB Conduction : fl_lib/Thermal/Thermal Elements/Conductive Heat Transfer  thermal_type=foundation.enum.ConstantVariableTabulated.Constant  wall_geometry=foundation.enum.ConductionWallGeometry.Planar  area=1 m^2  thickness=1 m  d_in=0.05 m  d_out=0.1 m  L=1 m  th_cond_min=10 W/(K*m)  th_cond=0.1 W/(m*K)  th_cond_TLU=[413, 401, 392, 383, 371, 357, 342] W/(K*m)  temp_TLU=[200, 273, 400, 600, 800, 1000, 1200] K  T_specify=off  T_priority=None  T=0 K  T_nominal_specify=off  T_nominal_value=1  T_nominal_unit=K  Q_specify=off  Q_priority=None  Q=0 J/s  Q_nominal_specify=off  Q_nominal_value=1  Q_nominal_unit=J/s
  WiA-WiB Convection : fl_lib/Thermal/Thermal Elements/Convective Heat Transfer  thermal_type=foundation.enum.constant_variable.constant  area=1 m^2  heat_tr_coeff=0.1 W/(m^2 * K)  min_heat_tr_coeff=1e-3 W/(K*m^2)  T_specify=off  T_priority=None  T=0 K  T_nominal_specify=off  T_nominal_value=1  T_nominal_unit=K  Q_specify=off  Q_priority=None  Q=0 J/s  Q_nominal_specify=off  Q_nominal_value=1  Q_nominal_unit=J/s
  WiA-WiC Conduction : fl_lib/Thermal/Thermal Elements/Conductive Heat Transfer  thermal_type=foundation.enum.ConstantVariableTabulated.Constant  wall_geometry=foundation.enum.ConductionWallGeometry.Planar  area=1 m^2  thickness=1 m  d_in=0.05 m  d_out=0.1 m  L=1 m  th_cond_min=10 W/(K*m)  th_cond=0.1 W/(m*K)  th_cond_TLU=[413, 401, 392, 383, 371, 357, 342] W/(K*m)  temp_TLU=[200, 273, 400, 600, 800, 1000, 1200] K  T_specify=off  T_priority=None  T=0 K  T_nominal_specify=off  T_nominal_value=1  T_nominal_unit=K  Q_specify=off  Q_priority=None  Q=0 J/s  Q_nominal_specify=off  Q_nominal_value=1  Q_nominal_unit=J/s
  WiA-WiC Convection : fl_lib/Thermal/Thermal Elements/Convective Heat Transfer  thermal_type=foundation.enum.constant_variable.constant  area=1 m^2  heat_tr_coeff=0.1 W/(m^2 * K)  min_heat_tr_coeff=1e-3 W/(K*m^2)  T_specify=off  T_priority=None  T=0 K  T_nominal_specify=off  T_nominal_value=1  T_nominal_unit=K  Q_specify=off  Q_priority=None  Q=0 J/s  Q_nominal_specify=off  Q_nominal_value=1  Q_nominal_unit=J/s
  WiB-Amb Convection : fl_lib/Thermal/Thermal Elements/Convective Heat Transfer  thermal_type=foundation.enum.constant_variable.constant  area=1 m^2  heat_tr_coeff=0.1 W/(m^2 * K)  min_heat_tr_coeff=1e-3 W/(K*m^2)  T_specify=off  T_priority=None  T=0 K  T_nominal_specify=off  T_nominal_value=1  T_nominal_unit=K  Q_specify=off  Q_priority=None  Q=0 J/s  Q_nominal_specify=off  Q_nominal_value=1  Q_nominal_unit=J/s
  WiB-Rot Convection : fl_lib/Thermal/Thermal Elements/Convective Heat Transfer  thermal_type=foundation.enum.constant_variable.constant  area=1 m^2  heat_tr_coeff=0.1 W/(m^2 * K)  min_heat_tr_coeff=1e-3 W/(K*m^2)  T_specify=off  T_priority=None  T=0 K  T_nominal_specify=off  T_nominal_value=1  T_nominal_unit=K  Q_specify=off  Q_priority=None  Q=0 J/s  Q_nominal_specify=off  Q_nominal_value=1  Q_nominal_unit=J/s
  WiB-WiC Conduction : fl_lib/Thermal/Thermal Elements/Conductive Heat Transfer  thermal_type=foundation.enum.ConstantVariableTabulated.Constant  wall_geometry=foundation.enum.ConductionWallGeometry.Planar  area=1 m^2  thickness=1 m  d_in=0.05 m  d_out=0.1 m  L=1 m  th_cond_min=10 W/(K*m)  th_cond=0.1 W/(m*K)  th_cond_TLU=[413, 401, 392, 383, 371, 357, 342] W/(K*m)  temp_TLU=[200, 273, 400, 600, 800, 1000, 1200] K  T_specify=off  T_priority=None  T=0 K  T_nominal_specify=off  T_nominal_value=1  T_nominal_unit=K  Q_specify=off  Q_priority=None  Q=0 J/s  Q_nominal_specify=off  Q_nominal_value=1  Q_nominal_unit=J/s
  WiB-WiC Convection : fl_lib/Thermal/Thermal Elements/Convective Heat Transfer  thermal_type=foundation.enum.constant_variable.constant  area=1 m^2  heat_tr_coeff=0.1 W/(m^2 * K)  min_heat_tr_coeff=1e-3 W/(K*m^2)  T_specify=off  T_priority=None  T=0 K  T_nominal_specify=off  T_nominal_value=1  T_nominal_unit=K  Q_specify=off  Q_priority=None  Q=0 J/s  Q_nominal_specify=off  Q_nominal_value=1  Q_nominal_unit=J/s
  WiC-Amb Convection : fl_lib/Thermal/Thermal Elements/Convective Heat Transfer  thermal_type=foundation.enum.constant_variable.constant  area=1 m^2  heat_tr_coeff=0.1 W/(m^2 * K)  min_heat_tr_coeff=1e-3 W/(K*m^2)  T_specify=off  T_priority=None  T=0 K  T_nominal_specify=off  T_nominal_value=1  T_nominal_unit=K  Q_specify=off  Q_priority=None  Q=0 J/s  Q_nominal_specify=off  Q_nominal_value=1  Q_nominal_unit=J/s
  WiC-Rot Convection : fl_lib/Thermal/Thermal Elements/Convective Heat Transfer  thermal_type=foundation.enum.constant_variable.constant  area=1 m^2  heat_tr_coeff=0.1 W/(m^2 * K)  min_heat_tr_coeff=1e-3 W/(K*m^2)  T_specify=off  T_priority=None  T=0 K  T_nominal_specify=off  T_nominal_value=1  T_nominal_unit=K  Q_specify=off  Q_priority=None  Q=0 J/s  Q_nominal_specify=off  Q_nominal_value=1  Q_nominal_unit=J/s
  Rotor : PMIOPort  Side=Left
  Winding C : PMIOPort  Port=2  Side=Right
  Winding B : PMIOPort  Port=3  Side=Right
  Winding A : PMIOPort  Port=4  Side=Right
  Env : PMIOPort  Port=5  Side=Left
  T : Outport
  wires:
  [TR2] -> Bus Creator/4  "TR"
  [TC2] -> Bus Creator/3  "TC"
  [TB2] -> Bus Creator/2  "TB"
  [TA2] -> Bus Creator/1  "TA"
  Bus Creator/1 -> T/1
  connections:
  Sensing Temperature Rot/LConn1 -- Rotor/RConn1 -- WiC-Rot Convection/LConn1 -- WiB-Rot Convection/LConn1 -- WiA-Rot Convection/LConn1
  WiA-Rot Convection/RConn1 -- WiA-WiC Conduction/RConn1 -- WiA-WiC Convection/RConn1 -- WiA-WiB Convection/LConn1 -- WiA-WiB Conduction/LConn1 -- WiA-Amb Convection/LConn1 -- Connection Label/LConn1 -- Sensing Temperature WiA/LConn1 -- Winding A/RConn1
  WiA-WiB Convection/RConn1 -- WiA-WiB Conduction/RConn1 -- WiB-Amb Convection/LConn1 -- Sensing Temperature WiB/LConn1 -- WiB-Rot Convection/RConn1 -- Winding B/RConn1 -- Connection Label3/LConn1 -- WiB-WiC Conduction/LConn1 -- WiB-WiC Convection/LConn1
  WiC-Rot Convection/RConn1 -- Winding C/RConn1 -- WiB-WiC Conduction/RConn1 -- WiB-WiC Convection/RConn1 -- WiC-Amb Convection/LConn1 -- Connection Label8/LConn1 -- WiA-WiC Convection/LConn1 -- WiA-WiC Conduction/LConn1 -- Sensing Temperature WiC/LConn1
  WiA-Amb Convection/RConn1 -- WiC-Amb Convection/RConn1 -- Env/RConn1 -- Connection Label4/LConn1 -- WiB-Amb Convection/RConn1

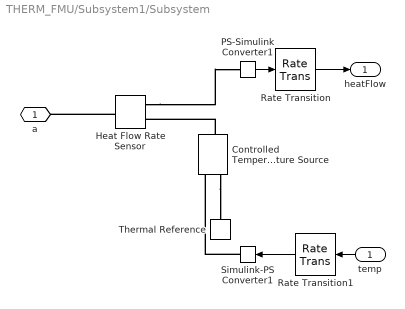
== system THERM_FMU/Subsystem1/Subsystem ==
  temp : Inport  SampleTime=TsTHERMAL
  Controlled Temperature Source : fl_lib/Thermal/Thermal Sources/Controlled Temperature Source
  Heat Flow Rate Sensor : fl_lib/Thermal/Thermal Sensors/Heat Flow Rate Sensor
  PS-Simulink Converter1 : nesl_utility/PS-Simulink Converter  PhysicalDomain=network_engine_domain  SubClassName=ps_output  LeftPortType=input  RightPortType=output  PseudoPeriodic=off  Frequencies=[]  VectorFormat=1-D array  Unit=inherit  AffineConversion=off
  Rate Transition : RateTransition  Deterministic=off  OutPortSampleTime=TsELEC
  Rate Transition1 : RateTransition  Deterministic=off  InitialCondition=323.15  OutPortSampleTime=TsTHERMAL
  Simulink-PS Converter1 : nesl_utility/Simulink-PS Converter  PhysicalDomain=network_engine_domain  SubClassName=ps_input  LeftPortType=input  RightPortType=output  PseudoPeriodic=off  Frequencies=[]  NoiseDistribution=none  NoiseParameters=[]  Unit=K  AffineConversion=off  FilteringAndDerivatives=provide  SimscapeFilterOrder=1  InputFilterTimeConstant=0.001  UdotUserProvided=0
  Thermal Reference : fl_lib/Thermal/Thermal Elements/Thermal Reference
  a : PMIOPort  Side=Left
  heatFlow : Outport  SampleTime=TsELEC
  wires:
  PS-Simulink Converter1/1 -> Rate Transition/1
  Rate Transition1/1 -> Simulink-PS Converter1/1
  temp/1 -> Rate Transition1/1
  Rate Transition/1 -> heatFlow/1
  connections:
  Heat Flow Rate Sensor/LConn1 -- a/RConn1
  Controlled Temperature Source/LConn1 -- Heat Flow Rate Sensor/RConn2
  Simulink-PS Converter1/RConn1 -- Controlled Temperature Source/RConn1
  Controlled Temperature Source/RConn2 -- Thermal Reference/LConn1
  Heat Flow Rate Sensor/RConn1 -- PS-Simulink Converter1/LConn1

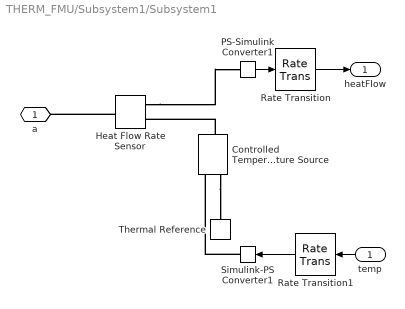
== system THERM_FMU/Subsystem1/Subsystem1 ==
  temp : Inport  SampleTime=TsTHERMAL
  Controlled Temperature Source : fl_lib/Thermal/Thermal Sources/Controlled Temperature Source
  Heat Flow Rate Sensor : fl_lib/Thermal/Thermal Sensors/Heat Flow Rate Sensor
  PS-Simulink Converter1 : nesl_utility/PS-Simulink Converter  PhysicalDomain=network_engine_domain  SubClassName=ps_output  LeftPortType=input  RightPortType=output  PseudoPeriodic=off  Frequencies=[]  VectorFormat=1-D array  Unit=inherit  AffineConversion=off
  Rate Transition : RateTransition  Deterministic=off  OutPortSampleTime=TsELEC
  Rate Transition1 : RateTransition  Deterministic=off  InitialCondition=323.15  OutPortSampleTime=TsTHERMAL
  Simulink-PS Converter1 : nesl_utility/Simulink-PS Converter  PhysicalDomain=network_engine_domain  SubClassName=ps_input  LeftPortType=input  RightPortType=output  PseudoPeriodic=off  Frequencies=[]  NoiseDistribution=none  NoiseParameters=[]  Unit=K  AffineConversion=off  FilteringAndDerivatives=provide  SimscapeFilterOrder=1  InputFilterTimeConstant=0.001  UdotUserProvided=0
  Thermal Reference : fl_lib/Thermal/Thermal Elements/Thermal Reference
  a : PMIOPort  Side=Left
  heatFlow : Outport  SampleTime=TsELEC
  wires:
  Rate Transition/1 -> heatFlow/1
  temp/1 -> Rate Transition1/1
  Rate Transition1/1 -> Simulink-PS Converter1/1
  PS-Simulink Converter1/1 -> Rate Transition/1
  connections:
  Heat Flow Rate Sensor/RConn1 -- PS-Simulink Converter1/LConn1
  Controlled Temperature Source/RConn2 -- Thermal Reference/LConn1
  Simulink-PS Converter1/RConn1 -- Controlled Temperature Source/RConn1
  Controlled Temperature Source/LConn1 -- Heat Flow Rate Sensor/RConn2
  Heat Flow Rate Sensor/LConn1 -- a/RConn1

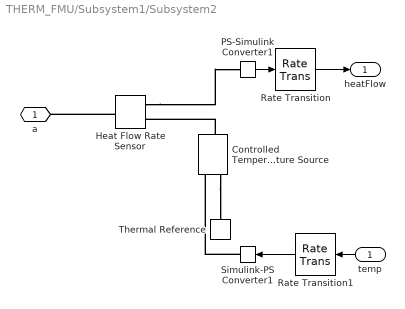
== system THERM_FMU/Subsystem1/Subsystem2 ==
  temp : Inport  SampleTime=TsTHERMAL
  Controlled Temperature Source : fl_lib/Thermal/Thermal Sources/Controlled Temperature Source
  Heat Flow Rate Sensor : fl_lib/Thermal/Thermal Sensors/Heat Flow Rate Sensor
  PS-Simulink Converter1 : nesl_utility/PS-Simulink Converter  PhysicalDomain=network_engine_domain  SubClassName=ps_output  LeftPortType=input  RightPortType=output  PseudoPeriodic=off  Frequencies=[]  VectorFormat=1-D array  Unit=inherit  AffineConversion=off
  Rate Transition : RateTransition  Deterministic=off  OutPortSampleTime=TsELEC
  Rate Transition1 : RateTransition  Deterministic=off  InitialCondition=323.15  OutPortSampleTime=TsTHERMAL
  Simulink-PS Converter1 : nesl_utility/Simulink-PS Converter  PhysicalDomain=network_engine_domain  SubClassName=ps_input  LeftPortType=input  RightPortType=output  PseudoPeriodic=off  Frequencies=[]  NoiseDistribution=none  NoiseParameters=[]  Unit=K  AffineConversion=off  FilteringAndDerivatives=provide  SimscapeFilterOrder=1  InputFilterTimeConstant=0.001  UdotUserProvided=0
  Thermal Reference : fl_lib/Thermal/Thermal Elements/Thermal Reference
  a : PMIOPort  Side=Left
  heatFlow : Outport  SampleTime=TsELEC
  wires:
  PS-Simulink Converter1/1 -> Rate Transition/1
  Rate Transition1/1 -> Simulink-PS Converter1/1
  temp/1 -> Rate Transition1/1
  Rate Transition/1 -> heatFlow/1
  connections:
  Heat Flow Rate Sensor/LConn1 -- a/RConn1
  Controlled Temperature Source/LConn1 -- Heat Flow Rate Sensor/RConn2
  Simulink-PS Converter1/RConn1 -- Controlled Temperature Source/RConn1
  Controlled Temperature Source/RConn2 -- Thermal Reference/LConn1
  Heat Flow Rate Sensor/RConn1 -- PS-Simulink Converter1/LConn1

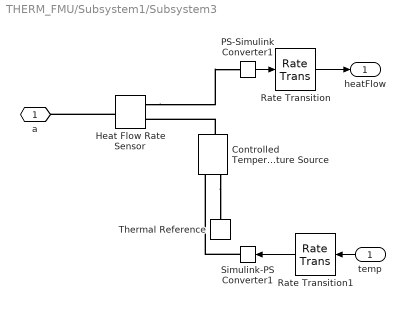
== system THERM_FMU/Subsystem1/Subsystem3 ==
  temp : Inport  SampleTime=TsTHERMAL
  Controlled Temperature Source : fl_lib/Thermal/Thermal Sources/Controlled Temperature Source
  Heat Flow Rate Sensor : fl_lib/Thermal/Thermal Sensors/Heat Flow Rate Sensor
  PS-Simulink Converter1 : nesl_utility/PS-Simulink Converter  PhysicalDomain=network_engine_domain  SubClassName=ps_output  LeftPortType=input  RightPortType=output  PseudoPeriodic=off  Frequencies=[]  VectorFormat=1-D array  Unit=inherit  AffineConversion=off
  Rate Transition : RateTransition  Deterministic=off  OutPortSampleTime=TsELEC
  Rate Transition1 : RateTransition  Deterministic=off  InitialCondition=323.15  OutPortSampleTime=TsTHERMAL
  Simulink-PS Converter1 : nesl_utility/Simulink-PS Converter  PhysicalDomain=network_engine_domain  SubClassName=ps_input  LeftPortType=input  RightPortType=output  PseudoPeriodic=off  Frequencies=[]  NoiseDistribution=none  NoiseParameters=[]  Unit=K  AffineConversion=off  FilteringAndDerivatives=provide  SimscapeFilterOrder=1  InputFilterTimeConstant=0.001  UdotUserProvided=0
  Thermal Reference : fl_lib/Thermal/Thermal Elements/Thermal Reference
  a : PMIOPort  Side=Left
  heatFlow : Outport  SampleTime=TsELEC
  wires:
  Rate Transition/1 -> heatFlow/1
  temp/1 -> Rate Transition1/1
  Rate Transition1/1 -> Simulink-PS Converter1/1
  PS-Simulink Converter1/1 -> Rate Transition/1
  connections:
  Heat Flow Rate Sensor/RConn1 -- PS-Simulink Converter1/LConn1
  Controlled Temperature Source/RConn2 -- Thermal Reference/LConn1
  Simulink-PS Converter1/RConn1 -- Controlled Temperature Source/RConn1
  Controlled Temperature Source/LConn1 -- Heat Flow Rate Sensor/RConn2
  Heat Flow Rate Sensor/LConn1 -- a/RConn1

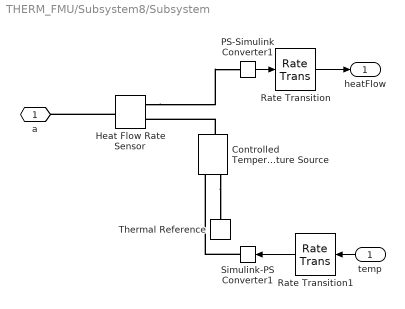
== system THERM_FMU/Subsystem8/Subsystem ==
  temp : Inport  SampleTime=TsTHERMAL
  Controlled Temperature Source : fl_lib/Thermal/Thermal Sources/Controlled Temperature Source
  Heat Flow Rate Sensor : fl_lib/Thermal/Thermal Sensors/Heat Flow Rate Sensor
  PS-Simulink Converter1 : nesl_utility/PS-Simulink Converter  PhysicalDomain=network_engine_domain  SubClassName=ps_output  LeftPortType=input  RightPortType=output  PseudoPeriodic=off  Frequencies=[]  VectorFormat=1-D array  Unit=inherit  AffineConversion=off
  Rate Transition : RateTransition  Deterministic=off  OutPortSampleTime=TsELEC
  Rate Transition1 : RateTransition  Deterministic=off  InitialCondition=323.15  OutPortSampleTime=TsTHERMAL
  Simulink-PS Converter1 : nesl_utility/Simulink-PS Converter  PhysicalDomain=network_engine_domain  SubClassName=ps_input  LeftPortType=input  RightPortType=output  PseudoPeriodic=off  Frequencies=[]  NoiseDistribution=none  NoiseParameters=[]  Unit=K  AffineConversion=off  FilteringAndDerivatives=provide  SimscapeFilterOrder=1  InputFilterTimeConstant=0.001  UdotUserProvided=0
  Thermal Reference : fl_lib/Thermal/Thermal Elements/Thermal Reference
  a : PMIOPort  Side=Left
  heatFlow : Outport  SampleTime=TsELEC
  wires:
  Rate Transition/1 -> heatFlow/1
  temp/1 -> Rate Transition1/1
  Rate Transition1/1 -> Simulink-PS Converter1/1
  PS-Simulink Converter1/1 -> Rate Transition/1
  connections:
  Heat Flow Rate Sensor/RConn1 -- PS-Simulink Converter1/LConn1
  Controlled Temperature Source/RConn2 -- Thermal Reference/LConn1
  Simulink-PS Converter1/RConn1 -- Controlled Temperature Source/RConn1
  Controlled Temperature Source/LConn1 -- Heat Flow Rate Sensor/RConn2
  Heat Flow Rate Sensor/LConn1 -- a/RConn1
